simulink model "genSym"  (R2024b)
settings: Solver=VariableStepAuto  StartTime=0.0  StopTime=10.0  RelTol=1e-3
values from neighbouring files (symbols this model uses):
  x0 = zeros(18,1)    [LoadSimulation.m]    (also in Variables.sldd = 1.0 0.0 0.0 0.0 0.0 0.0 0.0 0.0 0.0 0.0 0.0 0.0 0.0 0.0 0.0 ; run_sim.m = zeros(12,1))
undefined symbols (not defined in the file or in its folder): DiscIntNeverNeededParam, linSys
settings Model: Creator=antho  LastModifiedBy=pplat

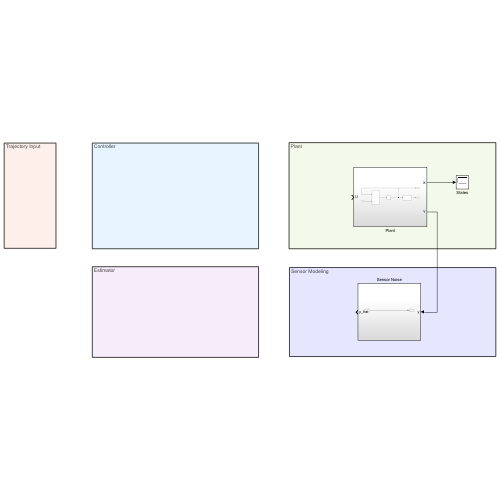
[thumbnail: Simulink's stored preview of the top-level diagram]
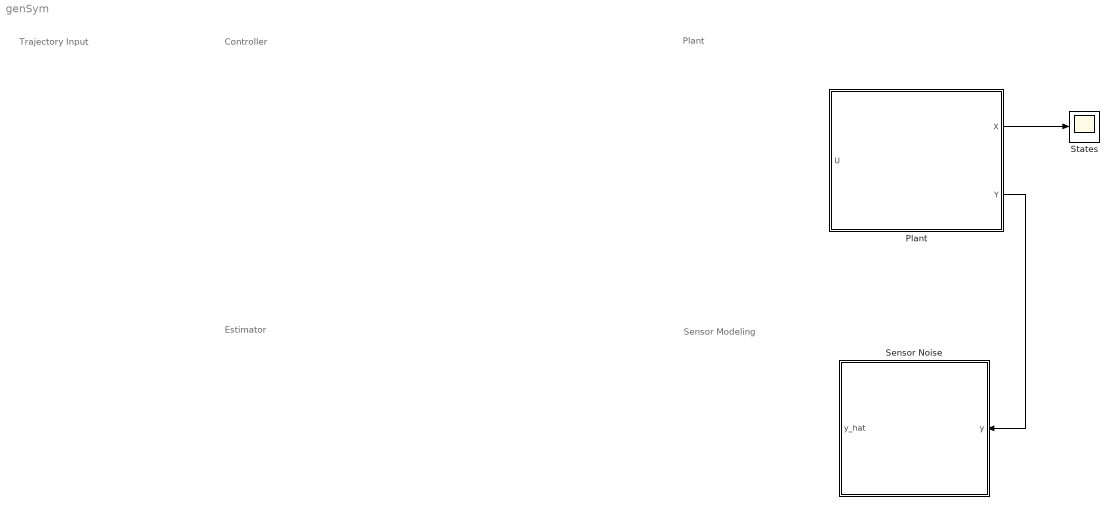
== system genSym ==
  note: Trajectory Input
  note: Estimator
  note: Controller
  note: Sensor Modeling
  note: Plant
  Plant : Subsystem
  Sensor Noise : Subsystem
  States : Scope
  wires:
  Plant/2(Y) -> Sensor Noise/1(y)
  Plant/1(X) -> States/1

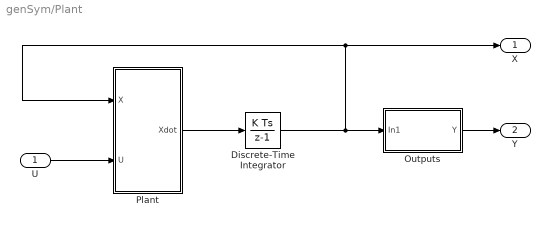
== system genSym/Plant ==
  U : Inport
  Discrete-Time Integrator : DiscreteIntegrator  InitialCondition=x0  SampleTime=-1  ICPrevOutput=DiscIntNeverNeededParam  ICPrevScaledInput=DiscIntNeverNeededParam
  Outputs : Subsystem
  Plant : MATLAB Function  TreatAsAtomicUnit=on
  X : Outport
  Y : Outport  Port=2
  wires:
  Discrete-Time Integrator/1 -> Outputs/1(In1), X/1, Plant/1(X)
  Plant/1(Xdot) -> Discrete-Time Integrator/1
  U/1 -> Plant/2(U)
  Outputs/1(Y) -> Y/1

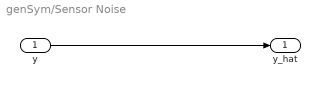
== system genSym/Sensor Noise ==
  y : Inport
  y_hat : Outport
  wires:
  y/1 -> y_hat/1

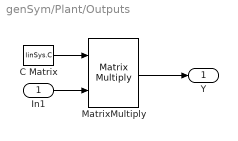
== system genSym/Plant/Outputs ==
  In1 : Inport
  C Matrix : Constant  Value=linSys.C
  MatrixMultiply : Product  Multiplication=Matrix(*)
  Y : Outport
  wires:
  MatrixMultiply/1 -> Y/1
  C Matrix/1 -> MatrixMultiply/1
  In1/1 -> MatrixMultiply/2

== matlab function genSym/Plant/Plant ==
  data: X input; Xdot output; U input
function Xdot = dynamics(X, U)

Xdot = plantfcn(X, U);
end
